simulink model "myproj"  (R2020a)
settings: Solver=VariableStepAuto  StartTime=0.0  StopTime=70  RelTol=1e-3
values from neighbouring files (symbols this model uses):
  b = 3.97e-6    (= 3.97e-06)    [run.m]
  g = 9.81    [run.m]
  GR = 2.5    [run.m]
  i_0 = 0    [run.m]
  J = 0.0001    [run.m]
  kb = 0.00574    [run.m]
  km = kb    (= 0.00574)    [run.m]
  L = 0.003    [run.m]
  m = 1.136    [run.m]
  Q = 0.37    [run.m]
  R = 0.141    [run.m]
  Rw = 3.2e-2    (= 0.032)    [run.m]
  tht_0 = 0    [run.m]
  tol = 1.0e-10    (= 1e-10)    [run.m]
  v_0 = 0    [run.m]
  wm_0 = 0    [run.m]
  wm_des = 275    [run.m]
  xp_0 = 0    [run.m]
libraries: simulink x1
settings Model: Creator=r_nazee  LastModifiedBy=r_nazee

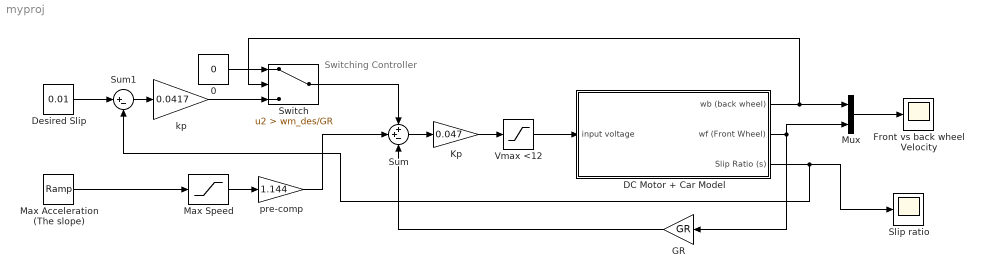
== system myproj ==
  note: Switching Controller
  0 : Constant  Value=0
  DC Motor + Car Model : Subsystem
  Desired Slip : Constant  Value=0.01
  Front vs back wheel Velocity : Scope
  GR : Gain  Gain=GR
  Kp : Gain  Gain=0.047
  Max Acceleration (The slope) : simulink/Sources/Ramp  slope=50  start=0  InitialOutput=0
  Max Speed : Saturate  UpperLimit=wm_des  LowerLimit=0
  Mux : Mux  Inputs=2
  "Slip ratio " : Scope
  Sum : Sum  Inputs=++-
  Sum1 : Sum  Inputs=|+-
  Switch : Switch  Criteria=u2 > Threshold  Threshold=wm_des/GR
  Vmax <12 : Saturate  UpperLimit=12  LowerLimit=0
  kp : Gain  Gain=0.0417
  pre-comp : Gain  Gain=1.144
  wires:
  DC Motor + Car Model/2(wf (Front Wheel)) -> GR/1, Mux/2
  GR/1 -> Sum/3
  Sum/1 -> Kp/1
  Kp/1 -> Vmax <12/1
  Max Acceleration (The slope)/1 -> Max Speed/1
  Max Speed/1 -> pre-comp/1
  pre-comp/1 -> Sum/2
  0/1 -> Switch/1
  Switch/1 -> Sum/1
  Desired Slip/1 -> Sum1/1
  Sum1/1 -> kp/1
  kp/1 -> Switch/3
  DC Motor + Car Model/1(wb (back wheel)) -> Switch/2, Mux/1
  Mux/1 -> Front vs back wheel Velocity/1
  DC Motor + Car Model/3(Slip Ratio (s)) -> Sum1/2, "Slip ratio "/1
  Vmax <12/1 -> DC Motor + Car Model/1(input voltage)

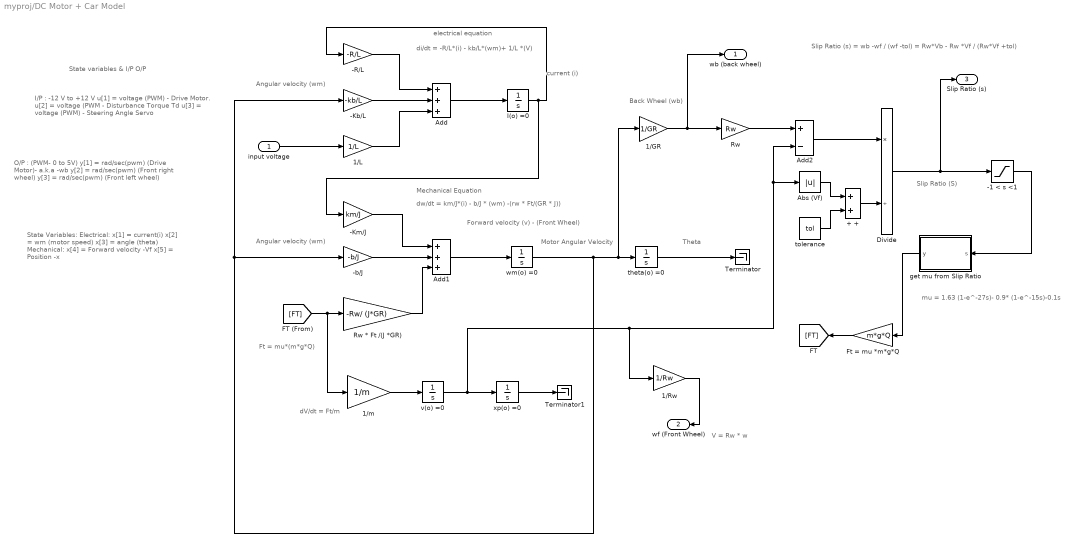
== system myproj/DC Motor + Car Model ==
  note: V = Rw * w
  note: mu = 1.63 (1-e^-27s)- 0.9* (1-e^-15s)-0.1s
  note: Slip Ratio (s) = wb -wf / (wf -tol) = Rw*Vb - Rw *Vf / (Rw*Vf +tol)
  note: Ft = mu*(m*g*Q)
  note: dV/dt = Ft/m
  note: Mechanical Equation
  note: dw/dt = km/J*(i) - b/J * (wm) -(rw * Ft/(GR * J))
  note: current (i)
  note: electrical equation
  note: di/dt = -R/L*(i) - kb/L*(wm)+ 1/L *(V)
  note: Slip Ratio (S)
  note: Forward velocity (v) - (Front Wheel)
  note: Back Wheel (wb)
  note: Angular velocity (wm)
  note: Angular velocity (wm)
  note: Motor Angular Velocity
  note: Theta
  note: State variables & I/P O/P
  note: I/P : -12 V to +12 V
      | u[1] = voltage (PWM) - Drive Motor.
      | u[2] = voltage (PWM - Disturbance Torque Td
      | u[3] = voltage (PWM) - Steering Angle Servo
  note: O/P : (PWM- 0 to 5V)
      |  y[1] = rad/sec(pwm) (Drive Motor)- a.k.a -wb
      |  y[2] = rad/sec(pwm) (Front right wheel)
      |  y[3] = rad/sec(pwm) (Front left wheel)
  note: State Variables:
      |
      | Electrical:
      | x[1] = current(i)
      | x[2] = wm (motor speed)
      | x[3] = angle (theta)
      |
      | Mechanical:
      | x[4] = Forward velocity -Vf
      | x[5] = Position -x
  input voltage : Inport
  + + : Sum
  -1 < s <1 : Saturate  UpperLimit=1  LowerLimit=-1
  -Kb/L : Gain  Gain=-kb/L
  -Km/J : Gain  Gain=km/J
  -R/L : Gain  Gain=-R/L
  -b/J : Gain  Gain=-b/J
  1/GR : Gain  Gain=1/GR
  1/L : Gain  Gain=1/L
  1/Rw : Gain  Gain=1/Rw
  1/m : Gain  Gain=1/m
  Abs (Vf) : Abs
  Add : Sum  Inputs=+++
  Add1 : Sum  Inputs=+++
  Add2 : Sum  Inputs=+-
  Divide : Product  Inputs=*/
  Ft = mu *m*g*Q : Gain  Gain=m*g*Q
  I(o) =0 : Integrator  InitialCondition=i_0
  Rw : Gain  Gain=Rw
  "Rw * Ft /(J *GR) " : Gain  Gain=-Rw/ (J*GR)
  Terminator : Terminator
  Terminator1 : Terminator
  get mu from Slip Ratio : MATLAB Function  TreatAsAtomicUnit=on
  theta(o) =0 : Integrator  InitialCondition=tht_0
  tolerance : Constant  Value=tol
  v(o) =0 : Integrator  InitialCondition=v_0
  wm(o) =0 : Integrator  InitialCondition=wm_0
  xp(o) =0 : Integrator  InitialCondition=xp_0
  wb (back wheel) : Outport
  wf (Front Wheel) : Outport  Port=2
  Slip Ratio (s) : Outport  Port=3
  wires:
  Add/1 -> I(o) =0/1
  Rw/1 -> Add2/1
  -R/L/1 -> Add/1
  I(o) =0/1 -> -Km/J/1, -R/L/1
  wm(o) =0/1 -> -b/J/1, -Kb/L/1, 1/GR/1, theta(o) =0/1
  1/GR/1 -> wb (back wheel)/1, Rw/1
  + +/1 -> Divide/2
  v(o) =0/1 -> 1/Rw/1, Abs (Vf)/1, Add2/2, xp(o) =0/1
  get mu from Slip Ratio/1(y) -> Ft = mu *m*g*Q/1
  [FT] -> 1/m/1, "Rw * Ft /(J *GR) "/1
  -Kb/L/1 -> Add/2
  -Km/J/1 -> Add1/1
  Add1/1 -> wm(o) =0/1
  -b/J/1 -> Add1/2
  input voltage/1 -> 1/L/1
  theta(o) =0/1 -> Terminator/1
  1/L/1 -> Add/3
  "Rw * Ft /(J *GR) "/1 -> Add1/3
  Abs (Vf)/1 -> + +/1
  Ft = mu *m*g*Q/1 -> [FT]
  1/m/1 -> v(o) =0/1
  Add2/1 -> Divide/1
  xp(o) =0/1 -> Terminator1/1
  Divide/1 -> Slip Ratio (s)/1, -1 < s <1/1
  tolerance/1 -> + +/2
  1/Rw/1 -> wf (Front Wheel)/1
  -1 < s <1/1 -> get mu from Slip Ratio/1(s)

== matlab function myproj/DC Motor + Car Model/get mu from Slip Ratio ==
  data: s input; y output
function y = fcn(s)

% slip ratio is already saturated
% only defined from -1 to 1
a1 = 1.63;
a2 =-0.9;
a3 =-0.1;

c1 =-27;
c2 =-15;

if(s<0)
    s= abs(s);
    mu = -(a1*(1-exp(c1*s))+a2*(1-exp(c2*s))+ a3*s);
else
    mu = a1*(1-exp(c1*s))+a2*(1-exp(c2*s))+ a3*s;
end
y = mu;
